simulink model "PMSM_Control"  (R2015b)
settings: Solver=FixedStepAuto  StartTime=0.0  StopTime=10  FixedStep=0.001  RelTol=1e-3
values from neighbouring files (symbols this model uses):
  c_drag_pro = c_drag*G1.^3*r.^3/G2.^3    [Control_Parameters.m]
  Den = [2*J_pro*L 2*J_pro*R 3*Kt^2]    [Control_Parameters.m]
  Den1 = [2*J_pro*L 2*Kv*L+2*J_pro*R 3*Kt^2+2*Kv*R]    [Control_Parameters.m]
  J_pro = (m*r^2+J_G2)*(G1/G2)^2 + J_G1    (= 0.281547798877)    [Control_Parameters.m]
  Kt = .07329    (= 0.07329)    [Control_Parameters.m]
  Kv = 0.001    [Control_Parameters.m]
  L = 4e-5    (= 4e-05)    [Control_Parameters.m]
  Num = [3*Kt]    [Control_Parameters.m]
  Num1 = [2*J_pro 2*Kv]    [Control_Parameters.m]
  R = .013/2    (= 0.0065)    [Control_Parameters.m]
undefined symbols (not defined in the file or in its folder): sigbuilder_block
libraries: simulink x5
settings Model: Creator=Morten  LastModifiedBy=Morten

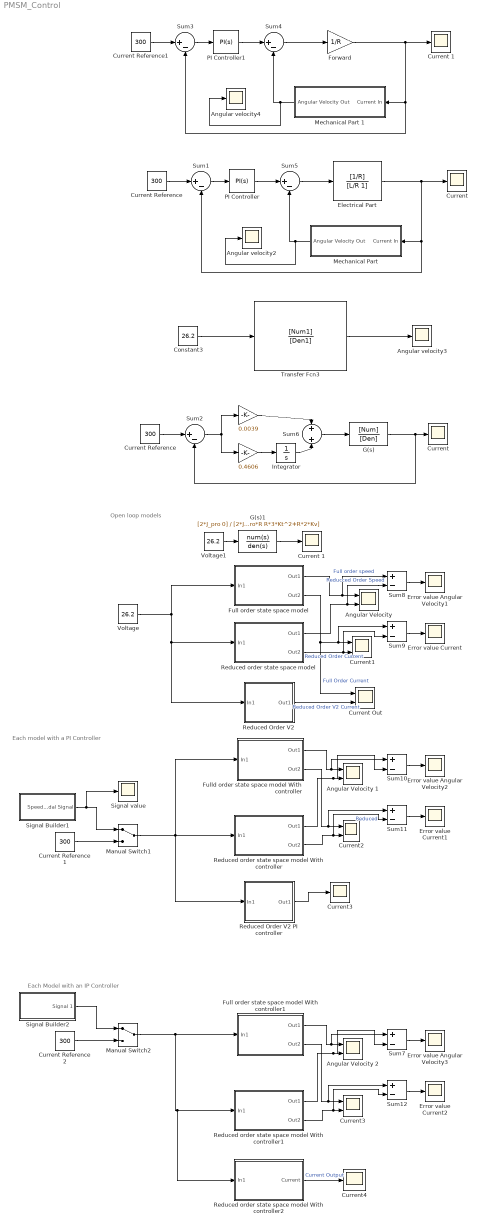
== system PMSM_Control ==
  note: Open loop models
  note: Each model with a PI Controller
  note: Each Model with an IP Controller
  " Current3" : Scope
  " " : Gain  Gain=0.4606
  " " : Gain  Gain=0.0039
  Angular Velocity 1 : Scope  NumInputPorts=2
  Angular Velocity 2 : Scope  NumInputPorts=2
  "Angular Velocity  " : Scope  NumInputPorts=2
  Angular velocity2 : Scope
  Angular velocity3 : Scope
  Angular velocity4 : Scope
  Constant3 : Constant  Value=26.2
  Current Out : Scope  NumInputPorts=2
  Current Reference : Constant  Value=300
  "Current Reference " : Constant  Value=300
  Current Reference 1 : Constant  Value=300
  Current Reference 2 : Constant  Value=300
  Current Reference1 : Constant  Value=300
  Current {,,1,1} (4 alike) : Scope
  Current1 : Scope  NumInputPorts=2
  Current2 : Scope  NumInputPorts=2
  Current3 : Scope  NumInputPorts=2
  Current4 : Scope
  Electrical Part : TransferFcn  Numerator=[1/R]  Denominator=[L/R 1]
  Error value Angular Velocity1 : Scope
  Error value Angular Velocity2 : Scope
  Error value Angular Velocity3 : Scope
  Error value Current : Scope
  Error value Current1 : Scope
  Error value Current2 : Scope
  Forward : Gain  Gain=1/R
  Full order state space model : Subsystem
  Full order state space model With controller1 : Subsystem
  Fulld order state space model With controller : Subsystem
  G(s) : TransferFcn  Numerator=[Num]  Denominator=[Den]
  G(s)1 : TransferFcn  Numerator=[2*J_pro 0]  Denominator=[2*J_pro*R R*3*Kt^2+R*2*Kv]
  Integrator : Integrator
  Manual Switch1 : ManualSwitch
  Manual Switch2 : ManualSwitch
  "Mechanical Part " : Subsystem
  Mechanical Part 1 : Subsystem
  PI Controller : simulink/Continuous/PID Controller  Controller=PI  TimeDomain=Continuous-time  SampleTime=-1  IntegratorMethod=Forward Euler  FilterMethod=Forward Euler  Form=Parallel  UseFilter=on  ControllerParametersSource=internal  P=0.0039  I=0.4606  D=0  N=100  InitialConditionSource=internal  InitialConditionForIntegrator=0  InitialConditionForFilter=0  ExternalReset=none  LimitOutput=off  UpperSaturationLimit=inf  LowerSaturationLimit=-inf  LinearizeAsGain=on  AntiWindupMode=none  Kb=1  TrackingMode=off  Kt=1  PParamMin=[]  PParamMax=[]  IParamMin=[]  IParamMax=[]  DParamMin=[]  DParamMax=[]  NParamMin=[]  NParamMax=[]  KbParamMin=[]  KbParamMax=[]  KtParamMin=[]  KtParamMax=[]  POutMin=[]  POutMax=[]  IOutMin=[]  IOutMax=[]  DOutMin=[]  DOutMax=[]  NOutMin=[]  NOutMax=[]  KbOutMin=[]  KbOutMax=[]  KtOutMin=[]  KtOutMax=[]  IntegratorOutMin=[]  IntegratorOutMax=[]  FilterOutMin=[]  FilterOutMax=[]  SumOutMin=[]  SumOutMax=[]  SumI1OutMin=[]  SumI1OutMax=[]  SumI2OutMin=[]  SumI2OutMax=[]  SumI3OutMin=[]  SumI3OutMax=[]  SumDOutMin=[]  SumDOutMax=[]  SaturationOutMin=[]  SaturationOutMax=[]  IntegratorContinuousStateAttributes=''  IntegratorStateMustResolveToSignalObject=off  IntegratorRTWStateStorageClass=Auto  FilterContinuousStateAttributes=''  FilterStateMustResolveToSignalObject=off  FilterRTWStateStorageClass=Auto  DifferentiatorICPrevScaledInput=0  DifferentiatorOutMin=[]  DifferentiatorOutMax=[]
  PI Controller1 : simulink/Continuous/PID Controller  Controller=PI  TimeDomain=Continuous-time  SampleTime=-1  IntegratorMethod=Forward Euler  FilterMethod=Forward Euler  Form=Parallel  UseFilter=on  ControllerParametersSource=internal  P=0.0039  I=0.4606  D=0  N=100  InitialConditionSource=internal  InitialConditionForIntegrator=0  InitialConditionForFilter=0  ExternalReset=none  LimitOutput=off  UpperSaturationLimit=inf  LowerSaturationLimit=-inf  LinearizeAsGain=on  AntiWindupMode=none  Kb=1  TrackingMode=off  Kt=1  PParamMin=[]  PParamMax=[]  IParamMin=[]  IParamMax=[]  DParamMin=[]  DParamMax=[]  NParamMin=[]  NParamMax=[]  KbParamMin=[]  KbParamMax=[]  KtParamMin=[]  KtParamMax=[]  POutMin=[]  POutMax=[]  IOutMin=[]  IOutMax=[]  DOutMin=[]  DOutMax=[]  NOutMin=[]  NOutMax=[]  KbOutMin=[]  KbOutMax=[]  KtOutMin=[]  KtOutMax=[]  IntegratorOutMin=[]  IntegratorOutMax=[]  FilterOutMin=[]  FilterOutMax=[]  SumOutMin=[]  SumOutMax=[]  SumI1OutMin=[]  SumI1OutMax=[]  SumI2OutMin=[]  SumI2OutMax=[]  SumI3OutMin=[]  SumI3OutMax=[]  SumDOutMin=[]  SumDOutMax=[]  SaturationOutMin=[]  SaturationOutMax=[]  IntegratorContinuousStateAttributes=''  IntegratorStateMustResolveToSignalObject=off  IntegratorRTWStateStorageClass=Auto  FilterContinuousStateAttributes=''  FilterStateMustResolveToSignalObject=off  FilterRTWStateStorageClass=Auto  DifferentiatorICPrevScaledInput=0  DifferentiatorOutMin=[]  DifferentiatorOutMax=[]
  Reduced Order V2 : Subsystem
  Reduced Order V2 PI controller : Subsystem
  Reduced order state space model : Subsystem
  Reduced order state space model With controller : Subsystem
  Reduced order state space model With controller1 : Subsystem
  Reduced order state space model With controller2 : Subsystem
  Signal Builder1 : Subsystem  Tag=STV Subsys  LoadFcn=sigbuilder_block('load');  StartFcn=sigbuilder_block('start');  StopFcn=sigbuilder_block('stop');  ClipboardFcn=sigbuilder_block('clipboard');  mask(Sigbuilder block){}
      mask help: Simulink:masks:SigbuilderBlock_MD
      mask init:
      | if ~strcmp(get_param(bdroot(gcbh),'SimulationStatus'),'stopped') tuvar = sigbuilder_block('maskInit'); end
      settings: CopyFcn=sigbuilder_block('copy');  DeleteFcn=sigbuilder_block('delete');  ModelCloseFcn=sigbuilder_block('modelClose');  PreSaveFcn=sigbuilder_block('preSave');  PauseFcn=sigbuilder_block('pause');  ContinueFcn=sigbuilder_block('continue');  NameChangeFcn=sigbuilder_block('namechange');  OpenFcn=sigbuilder_block('open',[595.8 225 550.8 361.2 ]);  CloseFcn=sigbuilder_block('close');
      mask Display: plot(0, 0, 100, 100,[2, 2, 32, 32, 2], [68, 8, 8, 68, 68],[32, 2], [38, 38], [32, 19, 2],[53, 60, 44], [32, 17, 17, 2],[16, 16, 31, 31]);txt = getActiveGroup(gcbh);text(2, 100, txt,'verticalAlignment', 'top');
  Signal Builder2 : Subsystem  Tag=STV Subsys  LoadFcn=sigbuilder_block('load');  StartFcn=sigbuilder_block('start');  StopFcn=sigbuilder_block('stop');  ClipboardFcn=sigbuilder_block('clipboard');  mask(Sigbuilder block){}
      mask help: Simulink:masks:SigbuilderBlock_MD
      mask init:
      | if ~strcmp(get_param(bdroot(gcbh),'SimulationStatus'),'stopped') tuvar = sigbuilder_block('maskInit'); end
      settings: CopyFcn=sigbuilder_block('copy');  DeleteFcn=sigbuilder_block('delete');  ModelCloseFcn=sigbuilder_block('modelClose');  PreSaveFcn=sigbuilder_block('preSave');  PauseFcn=sigbuilder_block('pause');  ContinueFcn=sigbuilder_block('continue');  NameChangeFcn=sigbuilder_block('namechange');  OpenFcn=sigbuilder_block('open',[445.2 789 550.8 400.2 ]);  CloseFcn=sigbuilder_block('close');
      mask Display: plot(0, 0, 100, 100,[2, 2, 32, 32, 2], [68, 8, 8, 68, 68],[32, 2], [38, 38], [32, 19, 2],[53, 60, 44], [32, 17, 17, 2],[16, 16, 31, 31]);txt = getActiveGroup(gcbh);text(2, 100, txt,'verticalAlignment', 'top');
  Signal value : Scope
  Sum{1..5} (5 alike) : Sum  Inputs=|+-
  Sum{7..12} (6 alike) : Sum  Inputs=+-
  Sum6 : Sum
  Transfer Fcn3 : TransferFcn  Numerator=[Num1]  Denominator=[Den1]
  Voltage : Constant  Value=26.2
  Voltage1 : Constant  Value=26.2
  wires:
  PI Controller/1 -> Sum5/1
  Sum1/1 -> PI Controller/1
  Current Reference/1 -> Sum1/1
  "Mechanical Part "/1(Angular Velocity Out) -> Angular velocity2/1, Sum5/2
  Sum5/1 -> Electrical Part/1
  Electrical Part/1 -> Sum1/2, "Mechanical Part "/1(Current In), "Current "/1
  Constant3/1 -> Transfer Fcn3/1
  Transfer Fcn3/1 -> Angular velocity3/1
  Sum2/1 -> " "/1, " "/1
  "Current Reference "/1 -> Sum2/1
  G(s)/1 -> Sum2/2, "Current "/1
  " "/1 -> Sum6/1
  " "/1 -> Integrator/1
  Integrator/1 -> Sum6/2
  Sum6/1 -> G(s)/1
  Signal Builder1/1(Speeder Pedal Signal) -> Signal value/1, Manual Switch1/1
  Current Reference 1/1 -> Manual Switch1/2
  Voltage/1 -> Full order state space model/1(In1), Reduced Order V2/1(In1), Reduced order state space model/1(In1)
  Reduced order state space model/1(Out1) -> Sum8/2, "Angular Velocity  "/2  "Reducced Order Speed"
  Manual Switch1/1 -> Fulld order state space model With controller/1(In1), Reduced Order V2 PI controller/1(In1), Reduced order state space model With controller/1(In1)
  Fulld order state space model With controller/1(Out1) -> Sum10/1, Angular Velocity 1/1
  Reduced order state space model With controller/1(Out1) -> Sum10/2, Angular Velocity 1/2
  Full order state space model/2(Out2) -> Current Out/1, Sum9/1, Current1/1  "Full Order Current"
  Reduced order state space model/2(Out2) -> Sum9/2, Current1/2  "Reduced Order Current"
  Fulld order state space model With controller/2(Out2) -> Current2/1, Sum11/1
  Reduced order state space model With controller/2(Out2) -> Sum11/2, Current2/2  "Reduced"
  Sum8/1 -> Error value Angular Velocity1/1
  Sum9/1 -> Error value Current/1
  Sum10/1 -> Error value Angular Velocity2/1
  Sum11/1 -> Error value Current1/1
  PI Controller1/1 -> Sum4/1
  Sum3/1 -> PI Controller1/1
  Current Reference1/1 -> Sum3/1
  Mechanical Part 1/1(Angular Velocity Out) -> Angular velocity4/1, Sum4/2
  Sum4/1 -> Forward/1
  Forward/1 -> Sum3/2, Mechanical Part 1/1(Current In), Current 1/1
  Voltage1/1 -> G(s)1/1
  G(s)1/1 -> Current 1/1
  Signal Builder2/1(Signal 1) -> Manual Switch2/1
  Current Reference 2/1 -> Manual Switch2/2
  Manual Switch2/1 -> Reduced order state space model With controller2/1(In1), Reduced order state space model With controller1/1(In1), Full order state space model With controller1/1(In1)
  Full order state space model With controller1/1(Out1) -> Sum7/1, Angular Velocity 2/1
  Reduced order state space model With controller1/1(Out1) -> Sum7/2, Angular Velocity 2/2
  Full order state space model With controller1/2(Out2) -> Current3/1, Sum12/1
  Reduced order state space model With controller1/2(Out2) -> Sum12/2, Current3/2
  Sum7/1 -> Error value Angular Velocity3/1
  Sum12/1 -> Error value Current2/1
  Reduced order state space model With controller2/1(Current) -> Current4/1  "Current Output"
  Reduced Order V2/1(Out1) -> Current Out/2  "Reduced Order V2 Current"
  Full order state space model/1(Out1) -> Sum8/1, "Angular Velocity  "/1  "Full order speed"
  Reduced Order V2 PI controller/1(Out1) -> " Current3"/1

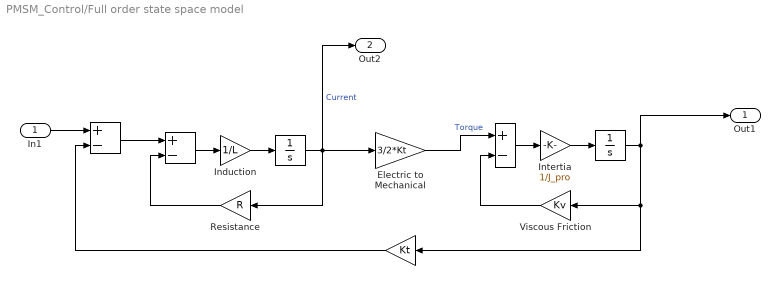
== system PMSM_Control/Full order state space model ==
  In1 : Inport
  "  " : Sum  Inputs=+-
  "   " : Sum  Inputs=+-
  "    " : Sum  Inputs=+-
  "                          " : Integrator
  "                            " : Gain  Gain=Kt
  "                                     " : Integrator
  Electric to Mechanical : Gain  Gain=3/2*Kt
  Induction : Gain  Gain=1/L
  Intertia : Gain  Gain=1/J_pro
  Resistance : Gain  Gain=R
  Viscous Friction : Gain  Gain=Kv
  Out1 : Outport
  Out2 : Outport  Port=2
  wires:
  "    "/1 -> Intertia/1
  "                          "/1 -> Out2/1, Resistance/1, Electric to Mechanical/1  "Current"
  Resistance/1 -> "   "/2
  "                            "/1 -> "  "/2
  Intertia/1 -> "                                     "/1
  "  "/1 -> "   "/1
  "   "/1 -> Induction/1
  Induction/1 -> "                          "/1
  In1/1 -> "  "/1
  "                                     "/1 -> Out1/1, "                            "/1, Viscous Friction/1
  Electric to Mechanical/1 -> "    "/1  "Torque"
  Viscous Friction/1 -> "    "/2

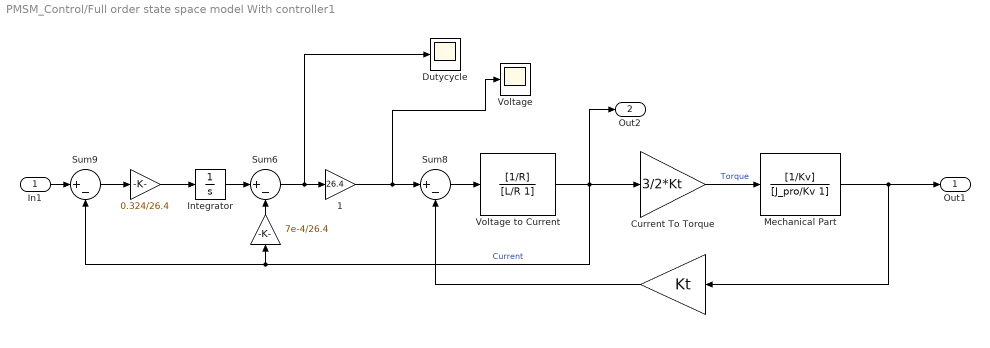
== system PMSM_Control/Full order state space model With controller1 ==
  In1 : Inport
  " " : Gain  Gain=0.324/26.4
  " " : Gain  Gain=7e-4/26.4
  " 1" : Gain  Gain=26.4
  "                " : Gain  Gain=Kt
  "Current To Torque " : Gain  Gain=3/2*Kt
  Dutycycle : Scope
  Integrator : Integrator
  "Mechanical Part " : TransferFcn  Numerator=[1/Kv]  Denominator=[J_pro/Kv 1]
  Sum6 : Sum  Inputs=|+-
  Sum8 : Sum  Inputs=|+-
  Sum9 : Sum  Inputs=|+-
  Voltage : Scope
  "Voltage to Current " : TransferFcn  Numerator=[1/R]  Denominator=[L/R 1]
  Out1 : Outport
  Out2 : Outport  Port=2
  wires:
  "                "/1 -> Sum8/2
  Sum8/1 -> "Voltage to Current "/1
  "Mechanical Part "/1 -> Out1/1, "                "/1
  In1/1 -> Sum9/1
  "Voltage to Current "/1 -> Out2/1, "Current To Torque "/1, Sum9/2, " "/1  "Current"
  "Current To Torque "/1 -> "Mechanical Part "/1  "Torque"
  Sum6/1 -> Dutycycle/1, " 1"/1
  " "/1 -> Sum6/2
  Integrator/1 -> Sum6/1
  " "/1 -> Integrator/1
  Sum9/1 -> " "/1
  " 1"/1 -> Voltage/1, Sum8/1

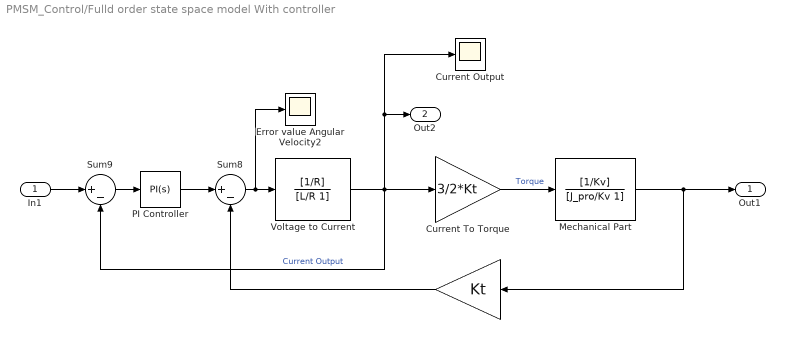
== system PMSM_Control/Fulld order state space model With controller ==
  In1 : Inport
  "                " : Gain  Gain=Kt
  "Current To Torque " : Gain  Gain=3/2*Kt
  Current Output : Scope
  Error value Angular Velocity2 : Scope
  "Mechanical Part " : TransferFcn  Numerator=[1/Kv]  Denominator=[J_pro/Kv 1]
  "PI Controller " : simulink/Continuous/PID Controller  Controller=PI  TimeDomain=Continuous-time  SampleTime=-1  IntegratorMethod=Forward Euler  FilterMethod=Forward Euler  Form=Parallel  UseFilter=on  ControllerParametersSource=internal  P=0.0111  I=1.7566  D=0  N=100  InitialConditionSource=internal  InitialConditionForIntegrator=0  InitialConditionForFilter=0  ExternalReset=none  LimitOutput=off  UpperSaturationLimit=inf  LowerSaturationLimit=-inf  LinearizeAsGain=on  AntiWindupMode=none  Kb=1  TrackingMode=off  Kt=1  PParamMin=[]  PParamMax=[]  IParamMin=[]  IParamMax=[]  DParamMin=[]  DParamMax=[]  NParamMin=[]  NParamMax=[]  KbParamMin=[]  KbParamMax=[]  KtParamMin=[]  KtParamMax=[]  POutMin=[]  POutMax=[]  IOutMin=[]  IOutMax=[]  DOutMin=[]  DOutMax=[]  NOutMin=[]  NOutMax=[]  KbOutMin=[]  KbOutMax=[]  KtOutMin=[]  KtOutMax=[]  IntegratorOutMin=[]  IntegratorOutMax=[]  FilterOutMin=[]  FilterOutMax=[]  SumOutMin=[]  SumOutMax=[]  SumI1OutMin=[]  SumI1OutMax=[]  SumI2OutMin=[]  SumI2OutMax=[]  SumI3OutMin=[]  SumI3OutMax=[]  SumDOutMin=[]  SumDOutMax=[]  SaturationOutMin=[]  SaturationOutMax=[]  IntegratorContinuousStateAttributes=''  IntegratorStateMustResolveToSignalObject=off  IntegratorRTWStateStorageClass=Auto  FilterContinuousStateAttributes=''  FilterStateMustResolveToSignalObject=off  FilterRTWStateStorageClass=Auto  DifferentiatorICPrevScaledInput=0  DifferentiatorOutMin=[]  DifferentiatorOutMax=[]
  Sum8 : Sum  Inputs=|+-
  Sum9 : Sum  Inputs=|+-
  "Voltage to Current " : TransferFcn  Numerator=[1/R]  Denominator=[L/R 1]
  Out1 : Outport
  Out2 : Outport  Port=2
  wires:
  "                "/1 -> Sum8/2
  Sum8/1 -> Error value Angular Velocity2/1, "Voltage to Current "/1
  "Mechanical Part "/1 -> Out1/1, "                "/1
  In1/1 -> Sum9/1
  "Voltage to Current "/1 -> Current Output/1, Out2/1, "Current To Torque "/1, Sum9/2  "Current Output"
  "Current To Torque "/1 -> "Mechanical Part "/1  "Torque"
  "PI Controller "/1 -> Sum8/1
  Sum9/1 -> "PI Controller "/1

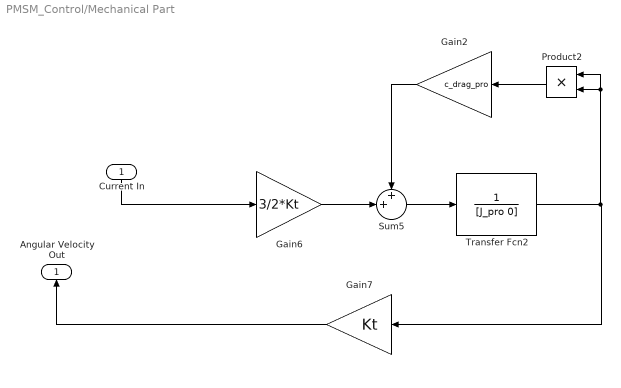
== system PMSM_Control/Mechanical Part  ==
  Current In : Inport
  Gain2 : Gain  Gain=c_drag_pro
  Gain6 : Gain  Gain=3/2*Kt
  Gain7 : Gain  Gain=Kt
  Product2 : Product
  Sum5 : Sum  Inputs=++|
  Transfer Fcn2 : TransferFcn  Denominator=[J_pro 0]
  Angular Velocity Out : Outport
  wires:
  Gain6/1 -> Sum5/2
  Transfer Fcn2/1 -> Product2/2, Product2/1, Gain7/1
  Gain2/1 -> Sum5/1
  Sum5/1 -> Transfer Fcn2/1
  Product2/1 -> Gain2/1
  Gain7/1 -> Angular Velocity Out/1
  Current In/1 -> Gain6/1

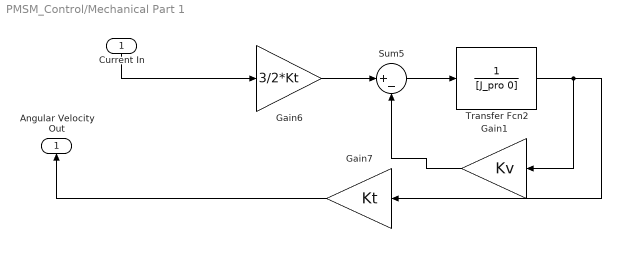
== system PMSM_Control/Mechanical Part 1 ==
  Current In : Inport
  Gain1 : Gain  Gain=Kv
  Gain6 : Gain  Gain=3/2*Kt
  Gain7 : Gain  Gain=Kt
  Sum5 : Sum  Inputs=|+-
  Transfer Fcn2 : TransferFcn  Denominator=[J_pro 0]
  Angular Velocity Out : Outport
  wires:
  Transfer Fcn2/1 -> Gain1/1, Gain7/1
  Sum5/1 -> Transfer Fcn2/1
  Gain7/1 -> Angular Velocity Out/1
  Current In/1 -> Gain6/1
  Gain1/1 -> Sum5/2
  Gain6/1 -> Sum5/1

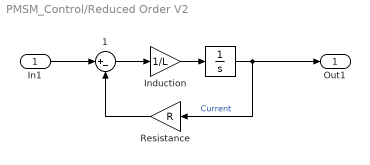
== system PMSM_Control/Reduced Order V2 ==
  In1 : Inport
  "               " : Integrator
  "     1" : Sum  Inputs=|+-
  "Induction  " : Gain  Gain=1/L
  "Resistance  " : Gain  Gain=R
  Out1 : Outport
  wires:
  "Induction  "/1 -> "               "/1
  "               "/1 -> Out1/1, "Resistance  "/1  "Current"
  "Resistance  "/1 -> "     1"/2
  In1/1 -> "     1"/1
  "     1"/1 -> "Induction  "/1

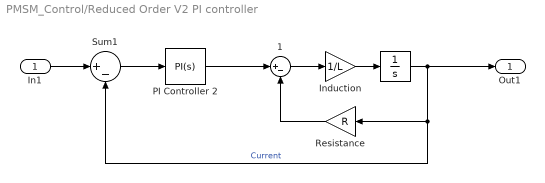
== system PMSM_Control/Reduced Order V2 PI controller ==
  In1 : Inport
  "               " : Integrator
  "     1" : Sum  Inputs=|+-
  "Induction  " : Gain  Gain=1/L
  PI Controller 2 : simulink/Continuous/PID Controller  Controller=PI  TimeDomain=Continuous-time  SampleTime=-1  IntegratorMethod=Forward Euler  FilterMethod=Forward Euler  Form=Parallel  UseFilter=on  ControllerParametersSource=internal  P=7e-4  I=0.324  D=0  N=100  InitialConditionSource=internal  InitialConditionForIntegrator=0  InitialConditionForFilter=0  ExternalReset=none  LimitOutput=off  UpperSaturationLimit=inf  LowerSaturationLimit=-inf  LinearizeAsGain=on  AntiWindupMode=none  Kb=1  TrackingMode=off  Kt=1  PParamMin=[]  PParamMax=[]  IParamMin=[]  IParamMax=[]  DParamMin=[]  DParamMax=[]  NParamMin=[]  NParamMax=[]  KbParamMin=[]  KbParamMax=[]  KtParamMin=[]  KtParamMax=[]  POutMin=[]  POutMax=[]  IOutMin=[]  IOutMax=[]  DOutMin=[]  DOutMax=[]  NOutMin=[]  NOutMax=[]  KbOutMin=[]  KbOutMax=[]  KtOutMin=[]  KtOutMax=[]  IntegratorOutMin=[]  IntegratorOutMax=[]  FilterOutMin=[]  FilterOutMax=[]  SumOutMin=[]  SumOutMax=[]  SumI1OutMin=[]  SumI1OutMax=[]  SumI2OutMin=[]  SumI2OutMax=[]  SumI3OutMin=[]  SumI3OutMax=[]  SumDOutMin=[]  SumDOutMax=[]  SaturationOutMin=[]  SaturationOutMax=[]  IntegratorContinuousStateAttributes=''  IntegratorStateMustResolveToSignalObject=off  IntegratorRTWStateStorageClass=Auto  FilterContinuousStateAttributes=''  FilterStateMustResolveToSignalObject=off  FilterRTWStateStorageClass=Auto  DifferentiatorICPrevScaledInput=0  DifferentiatorOutMin=[]  DifferentiatorOutMax=[]
  "Resistance  " : Gain  Gain=R
  Sum1 : Sum  Inputs=|+-
  Out1 : Outport
  wires:
  "     1"/1 -> "Induction  "/1
  "Resistance  "/1 -> "     1"/2
  "               "/1 -> "Resistance  "/1, Sum1/2, Out1/1  "Current"
  "Induction  "/1 -> "               "/1
  PI Controller 2/1 -> "     1"/1
  In1/1 -> Sum1/1
  Sum1/1 -> PI Controller 2/1

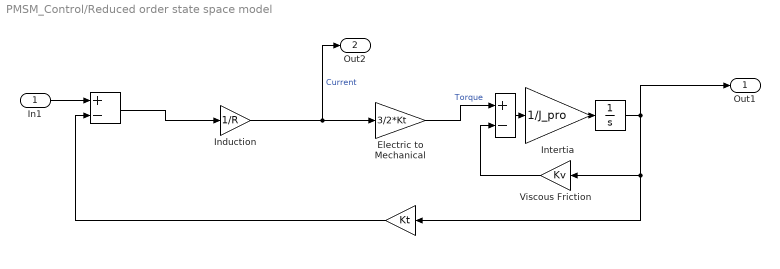
== system PMSM_Control/Reduced order state space model ==
  In1 : Inport
  "  " : Sum  Inputs=+-
  "    " : Sum  Inputs=+-
  "                            " : Gain  Gain=Kt
  "                                     " : Integrator
  Electric to Mechanical : Gain  Gain=3/2*Kt
  Induction : Gain  Gain=1/R
  Intertia : Gain  Gain=1/J_pro
  Viscous Friction : Gain  Gain=Kv
  Out1 : Outport
  Out2 : Outport  Port=2
  wires:
  "    "/1 -> Intertia/1
  Induction/1 -> Out2/1, Electric to Mechanical/1  "Current"
  "                            "/1 -> "  "/2
  Intertia/1 -> "                                     "/1
  "  "/1 -> Induction/1
  In1/1 -> "  "/1
  "                                     "/1 -> Out1/1, "                            "/1, Viscous Friction/1
  Electric to Mechanical/1 -> "    "/1  "Torque"
  Viscous Friction/1 -> "    "/2

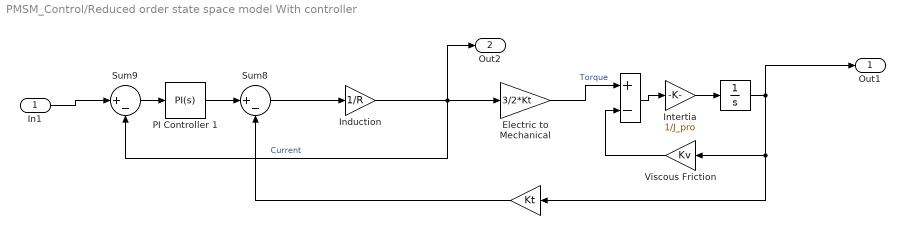
== system PMSM_Control/Reduced order state space model With controller ==
  In1 : Inport
  "    " : Sum  Inputs=+-
  "                            " : Gain  Gain=Kt
  "                                     " : Integrator
  Electric to Mechanical : Gain  Gain=3/2*Kt
  Induction : Gain  Gain=1/R
  Intertia : Gain  Gain=1/J_pro
  PI Controller 1 : simulink/Continuous/PID Controller  Controller=PI  TimeDomain=Continuous-time  SampleTime=-1  IntegratorMethod=Forward Euler  FilterMethod=Forward Euler  Form=Parallel  UseFilter=on  ControllerParametersSource=internal  P=0  I=2.96558030725913  D=0  N=100  InitialConditionSource=internal  InitialConditionForIntegrator=0  InitialConditionForFilter=0  ExternalReset=none  LimitOutput=off  UpperSaturationLimit=inf  LowerSaturationLimit=-inf  LinearizeAsGain=on  AntiWindupMode=none  Kb=1  TrackingMode=off  Kt=1  PParamMin=[]  PParamMax=[]  IParamMin=[]  IParamMax=[]  DParamMin=[]  DParamMax=[]  NParamMin=[]  NParamMax=[]  KbParamMin=[]  KbParamMax=[]  KtParamMin=[]  KtParamMax=[]  POutMin=[]  POutMax=[]  IOutMin=[]  IOutMax=[]  DOutMin=[]  DOutMax=[]  NOutMin=[]  NOutMax=[]  KbOutMin=[]  KbOutMax=[]  KtOutMin=[]  KtOutMax=[]  IntegratorOutMin=[]  IntegratorOutMax=[]  FilterOutMin=[]  FilterOutMax=[]  SumOutMin=[]  SumOutMax=[]  SumI1OutMin=[]  SumI1OutMax=[]  SumI2OutMin=[]  SumI2OutMax=[]  SumI3OutMin=[]  SumI3OutMax=[]  SumDOutMin=[]  SumDOutMax=[]  SaturationOutMin=[]  SaturationOutMax=[]  IntegratorContinuousStateAttributes=''  IntegratorStateMustResolveToSignalObject=off  IntegratorRTWStateStorageClass=Auto  FilterContinuousStateAttributes=''  FilterStateMustResolveToSignalObject=off  FilterRTWStateStorageClass=Auto  DifferentiatorICPrevScaledInput=0  DifferentiatorOutMin=[]  DifferentiatorOutMax=[]
  Sum8 : Sum  Inputs=|+-
  Sum9 : Sum  Inputs=|+-
  Viscous Friction : Gain  Gain=Kv
  Out1 : Outport
  Out2 : Outport  Port=2
  wires:
  "                                     "/1 -> Viscous Friction/1, "                            "/1, Out1/1
  Intertia/1 -> "                                     "/1
  Induction/1 -> Out2/1, Sum9/2, Electric to Mechanical/1  "Current"
  "    "/1 -> Intertia/1
  Sum8/1 -> Induction/1
  PI Controller 1/1 -> Sum8/1
  Sum9/1 -> PI Controller 1/1
  In1/1 -> Sum9/1
  "                            "/1 -> Sum8/2
  Electric to Mechanical/1 -> "    "/1  "Torque"
  Viscous Friction/1 -> "    "/2

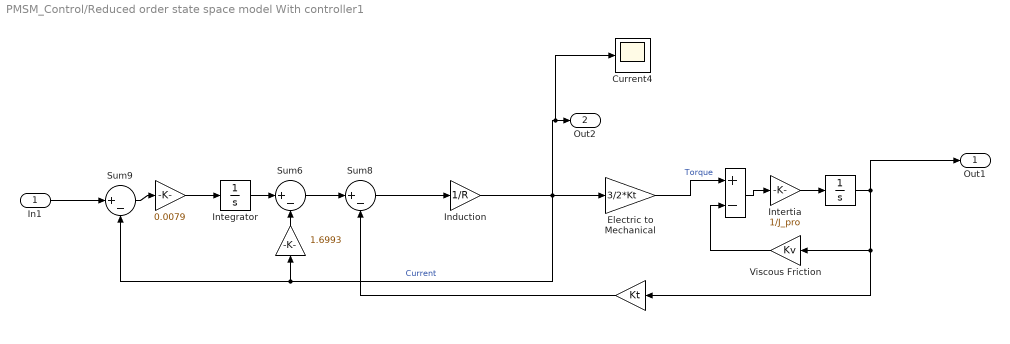
== system PMSM_Control/Reduced order state space model With controller1 ==
  In1 : Inport
  "    " : Sum  Inputs=+-
  " " : Gain  Gain=0.0079
  " " : Gain  Gain=1.6993
  "                            " : Gain  Gain=Kt
  "                                     " : Integrator
  Current4 : Scope
  Electric to Mechanical : Gain  Gain=3/2*Kt
  Induction : Gain  Gain=1/R
  Integrator : Integrator
  Intertia : Gain  Gain=1/J_pro
  Sum6 : Sum  Inputs=|+-
  Sum8 : Sum  Inputs=|+-
  Sum9 : Sum  Inputs=|+-
  Viscous Friction : Gain  Gain=Kv
  Out1 : Outport
  Out2 : Outport  Port=2
  wires:
  "                                     "/1 -> Viscous Friction/1, "                            "/1, Out1/1
  Intertia/1 -> "                                     "/1
  "    "/1 -> Intertia/1
  Sum8/1 -> Induction/1
  Sum6/1 -> Sum8/1
  In1/1 -> Sum9/1
  "                            "/1 -> Sum8/2
  Electric to Mechanical/1 -> "    "/1  "Torque"
  Viscous Friction/1 -> "    "/2
  Induction/1 -> Current4/1, Out2/1, " "/1, Sum9/2, Electric to Mechanical/1  "Current"
  " "/1 -> Sum6/2
  Integrator/1 -> Sum6/1
  " "/1 -> Integrator/1
  Sum9/1 -> " "/1

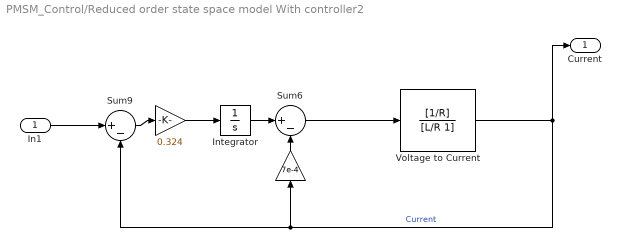
== system PMSM_Control/Reduced order state space model With controller2 ==
  In1 : Inport
  " " : Gain  Gain=0.324
  " " : Gain  Gain=7e-4
  Integrator : Integrator
  Sum6 : Sum  Inputs=|+-
  Sum9 : Sum  Inputs=|+-
  "Voltage to Current " : TransferFcn  Numerator=[1/R]  Denominator=[L/R 1]
  Current : Outport
  wires:
  Sum9/1 -> " "/1
  " "/1 -> Integrator/1
  Integrator/1 -> Sum6/1
  " "/1 -> Sum6/2
  "Voltage to Current "/1 -> Current/1, " "/1, Sum9/2  "Current"
  In1/1 -> Sum9/1
  Sum6/1 -> "Voltage to Current "/1

== system PMSM_Control/Signal Builder1 ==
  Demux : Demux  Tag=STV Demux  Outputs=1
  FromWs : FromWorkspace  Tag=STV FromWs  VariableName=tuvar  SampleTime=0
      SigBuilderData=|
      | common.afterFinalStr = 'Extrapolate'
      | common.sampleTime = 0
      | dataSet.timeRange = [0 10]
      | dataSet.name = 'Pedal Movement'
      | sbobj.Groups.Name = 'Pedal Movement'
      | sbobj.Groups.Signals.Name = 'Speeder Pedal Signal'
      | sbobj.Groups.Signals.XData = [0 0.1 4 6 6 10]
      | sbobj.Groups.Signals.YData = [0 300 300 1 0 0]
  Speeder Pedal Signal : Outport  Tag=STV Outport
  wires:
  Demux/1 -> Speeder Pedal Signal/1
  FromWs/1 -> Demux/1

== system PMSM_Control/Signal Builder2 ==
  Demux : Demux  Tag=STV Demux  Outputs=1
  FromWs : FromWorkspace  Tag=STV FromWs  VariableName=tuvar  SampleTime=0
      SigBuilderData=|
      | common.afterFinalStr = 'Extrapolate'
      | common.sampleTime = 0
      | dataSet.timeRange = [0 10]
      | dataSet.name = 'Group 1'
      | sbobj.Groups.Name = 'Group 1'
      | sbobj.Groups.Signals.Name = 'Signal 1'
      | sbobj.Groups.Signals.XData = [0 0.1 4 6 6 10]
      | sbobj.Groups.Signals.YData = [0 300 300 1 0 0]
  Signal 1 : Outport  Tag=STV Outport
  wires:
  Demux/1 -> Signal 1/1
  FromWs/1 -> Demux/1
